simulink model "TCT_long_wide_PVArray_PartialShading"  (R2016b)
settings: Solver=ode23tb  StartTime=0.0  StopTime=5  FixedStep=Ts_Power  RelTol=1e-4
PreLoadFcn:
  | Ts_Power=50e-6;
  | Slope_Vdc=1;
InitFcn:
  | Ts_Power=50e-6;
  | Tc=1e-5;%break algebraic loop time constant
  | BlockName=[gcs,'/PV cells 1-20'];
  | ModuleName=get_param(BlockName,'ModuleName');
  | Voc1=str2num(get_param(BlockName,'Voc'));
  | Nser1=str2num(get_param(BlockName,'Nser'));
  | Slope_Vdc=Nser1*Voc1;
StopFcn:
  | if exist('I','var') && exist('V','var')
  |    figure(1)
  |    clf
  |    n=find(I>=0);
  |    n=n(end);
  |    Vglobal=V(1:n);
  |    Iglobal=I(1:n);
  | 
  | 
  |    Pglobal=Vglobal.*Iglobal;
  |    n=find(Pglobal==max(Pglobal));
  |    Pmax=Pglobal(n);
  |    Vmp=Vglobal(n);
  |    Imp=Iglobal(n);
  | 
  | 
  |    subplot(211)
  |    plot(Vglobal, Iglobal,Vmp,Imp,'or')
  |    ylabel('Current (A)')
  |    title(sprintf('Global I-V & P-V characteristics\n %s' ,ModuleName))
  | 
  | 
  |    subplot(212)
  |    plot(Vglobal, Pglobal,Vmp,Pmax,'or')
  |    ylabel('Power (W)')
  |    xlabel('Voltage (V)')
  | end
libraries: powerlib x29, re_lib x25, simulink x1
Description:
  | Copyright 2008-2016 The MathWorks, Inc.
settings Model: Creator=MathWorks  LastModifiedBy=Gehaha
settings SolverCC: AlgebraicLoopSolver=LineSearch
settings DataIOCC: LimitDataPoints=on  SaveFormat=Array  SignalLoggingSaveFormat=ModelDataLogs
settings OptimizationCC: ExpressionDepthLimit=2147483647  LifeSpan=inf
settings DebuggingCC: UnderspecifiedInitializationDetection=Classic  MergeDetectMultiDrivingBlocksExec=none  SolverPrmCheckMsg=warning  FcnCallInpInsideContextMsg=warning  AllowSymbolicDim=off  StateNameClashWarn=warning  SFUnexpectedBacktrackingDiag=warning  SFNoUnconditionalDefaultTransitionDiag=warning  SFExecutionAtInitializationDiag=none
settings HardwareCC: ProdBitPerPointer=32  ProdBitPerSizeT=32  ProdBitPerPtrDiffT=32  ProdLargestAtomicFloat=None  ProdIntDivRoundTo=Undefined  ProdEndianess=Unspecified  ProdWordSize=32  ProdHWDeviceType=32-bit Generic
settings ModelReferenceCC: PropagateSignalLabelsOutOfModel=off
settings GRTTargetCC: TargetLangStandard=C89/C90 (ANSI)  GeneratePreprocessorConditionals=Disable all  CombineOutputUpdateFcns=off  GRTInterface=on
settings ConfigComp: CovMetricSettings=dw  CovHtmlReporting=on  CovSaveCumulativeToWorkspaceVar=on  CovSaveSingleToWorkspaceVar=on  CovExternalEMLEnable=off  CovSFcnEnable=off

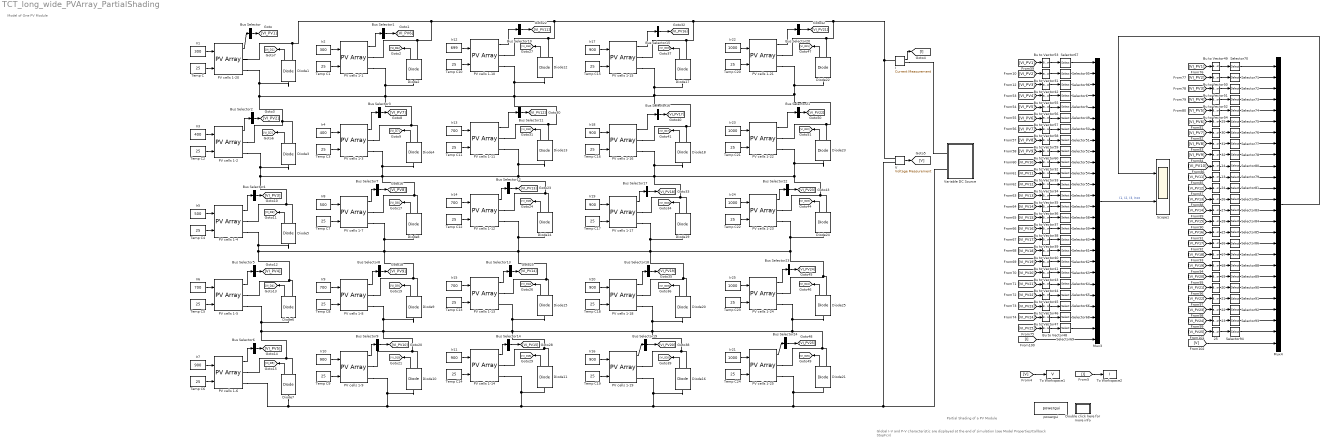
== system TCT_long_wide_PVArray_PartialShading ==
  note: Global I-V and P-V characteristic are displayed at the end of simulation
      | (see Model Properties/Callback StopFcn)
  note: Partial Shading of a PV Module
  note: Model of One PV Module
  {13..32} (20 alike) : BusToVector
  Bu to Vector{31..60} (30 alike) : BusToVector
  Bus Selector{,1..24} (25 alike) : BusSelector  OutputSignals=V_PV,I_PV  OutputAsBus=on
  Diode{1..25} (25 alike) : powerlib/Power Electronics/Diode  Ron=0.001  Lon=0  Vf=0.7  IC=0  UseSnubber=off  Rs=1e5*inf  Cs=inf  Measurements=on
  Double click here for more info : Subsystem
      settings: OpenFcn=showdemo(bdroot(gcb))
      mask Display: disp('?')
  I : powerlib/Measurements/Current Measurement  PhasorSimulation=off  OutputType=Complex  PSBequivalent=0
  Ir1 : Constant  Value=300
  Ir{7,10..11,16..20} (8 alike) : Constant  Value=900
  Ir12 : Constant  Value=699
  Ir{6,9,13..15} (5 alike) : Constant  Value=700
  Ir2 : Constant  Value=300
  Ir{21..25} (5 alike) : Constant  Value=1000
  Ir3 : Constant  Value=400
  Ir4 : Constant  Value=400
  Ir5 : Constant  Value=500
  Ir8 : Constant  Value=500
  Mux3 : Mux  Inputs=26
  Mux4 : Mux  Inputs=26
  PV cells 1-{1..25} (25 alike) : re_lib/Solar/PV Array  Npar=1  Nser=1  PlotType=array @ 25 deg.C & specified irradiances  S_vec="[ 1000  500  100 ]"  Temp_C_vec="[ 45 25  ]"  ModuleName=User-defined  PlotWhenSelected=off  Pm=83.2824  Ncell=60/3  Voc=37.92*20/60  Isc=8.62  Vm=30.96*20/60  Im=8.07  beta_Voc_pc=-0.33969  alpha_Isc_pc=0.063701  beta_Voc=-0.042937  alpha_Isc=0.005491  IL=8.6307  I0=1.4176e-10  nI=0.99132  Rsh=82.1161  Rs=0.098625  BAL=on  Tc=Tc  Tfilter=5e-5
  Scope1 : Scope  NumInputPorts=2
  Selector{6,9,49..69,95..96} (25 alike) : Selector  InputPortWidth=2  IndexOptions=Index vector (dialog)  Indices=[2]  OutputSizes=1
  Selector{70..94} (25 alike) : Selector  InputPortWidth=2  IndexOptions=Index vector (dialog)  Indices=[1]  OutputSizes=1
  Temp C{,1..24} (25 alike) : Constant  Value=25
  To Workspace1 : ToWorkspace  VariableName=V  SampleTime=1e-3
  To Workspace2 : ToWorkspace  VariableName=I  SampleTime=1e-3
  V : powerlib/Measurements/Voltage Measurement  PhasorSimulation=off  OutputType=Complex  PSBequivalent=0
  Variable DC Source : Subsystem
  powergui : powerlib/powergui  Priority=1  SimulationMode=Continuous  SolverType=Tustin/Backward Euler (TBE)  SampleTime=Ts_Power*0 + 20e-6  frequency=60  SPID=off  DisableSnubberDevices=on  DisableRonSwitches=off  DisableVfSwitches=off  SwTol=0  DisplayEquations=off  Interpol=off  ExternalGateDelay=off  methode=off  Ts=0  FunctionMessages=off  echomessages=off  HookPort=off  EnableUseOfTLC=off  x0status=blocks  frequencyindice=0  Pbase=100e6  ErrMax=1e-4  Iterations=50  UnitsV=kV  UnitsW=MW  buscounter=0  RestoreLinks=warning  ResistiveCurrentMeasurement=off  Frange=[0:2:500]  Ylog=off  Xlog=on  ShowGrid=off  save=off  variable=ZData  structure=0  ZoomFFT=on  StartTime=0.0  cycles=1  DisplayStyle=1  fundamental=60  FreqAxis=off  MaxFrequency=1000  frequencyindicesteady=1  RmsSteady=1  display=off
  wires:
  Ir1/1 -> PV cells 1-20/1
  Temp C/1 -> PV cells 1-20/2
  I/1 -> [I]
  V/1 -> [V]
  Diode1/1 -> [VI_D1]
  PV cells 1-20/1 -> Bus Selector/1
  Bus Selector/1 -> [VI_PV1]
  [V] -> To Workspace1/1
  [I] -> To Workspace2/1
  Ir2/1 -> PV cells 1-1/1
  Temp C1/1 -> PV cells 1-1/2
  Diode2/1 -> [VI_D6]
  PV cells 1-1/1 -> Bus Selector1/1
  Bus Selector1/1 -> [VI_PV6]
  Ir3/1 -> PV cells 1-2/1
  Temp C2/1 -> PV cells 1-2/2
  Diode3/1 -> [VI_D2]
  PV cells 1-2/1 -> Bus Selector2/1
  Bus Selector2/1 -> [VI_PV2]
  Ir4/1 -> PV cells 1-3/1
  Temp C3/1 -> PV cells 1-3/2
  Diode4/1 -> [VI_D7]
  PV cells 1-3/1 -> Bus Selector3/1
  Bus Selector3/1 -> [VI_PV7]
  Ir5/1 -> PV cells 1-4/1
  Temp C4/1 -> PV cells 1-4/2
  Diode5/1 -> [VI_D3]
  PV cells 1-4/1 -> Bus Selector4/1
  Bus Selector4/1 -> [VI_PV3]
  Ir6/1 -> PV cells 1-5/1
  Temp C5/1 -> PV cells 1-5/2
  Diode6/1 -> [VI_D4]
  PV cells 1-5/1 -> Bus Selector5/1
  Bus Selector5/1 -> [VI_PV4]
  Ir7/1 -> PV cells 1-6/1
  Temp C6/1 -> PV cells 1-6/2
  Diode7/1 -> [VI_D5]
  PV cells 1-6/1 -> Bus Selector6/1
  Bus Selector6/1 -> [VI_PV5]
  Ir8/1 -> PV cells 1-7/1
  Temp C7/1 -> PV cells 1-7/2
  Diode8/1 -> [VI_D8]
  PV cells 1-7/1 -> Bus Selector7/1
  Bus Selector7/1 -> [VI_PV8]
  Ir9/1 -> PV cells 1-8/1
  Temp C8/1 -> PV cells 1-8/2
  Diode9/1 -> [VI_D9]
  PV cells 1-8/1 -> Bus Selector8/1
  Bus Selector8/1 -> [VI_PV9]
  Ir10/1 -> PV cells 1-9/1
  Temp C9/1 -> PV cells 1-9/2
  Diode10/1 -> [VI_D10]
  PV cells 1-9/1 -> Bus Selector9/1
  Bus Selector9/1 -> [VI_PV10]
  Ir12/1 -> PV cells 1-10/1
  Temp C10/1 -> PV cells 1-10/2
  Diode12/1 -> [VI_D11]
  PV cells 1-10/1 -> Bus Selector10/1
  Bus Selector10/1 -> [VI_PV11]
  Ir13/1 -> PV cells 1-11/1
  Temp C11/1 -> PV cells 1-11/2
  Diode13/1 -> [VI_D12]
  PV cells 1-11/1 -> Bus Selector11/1
  Bus Selector11/1 -> [VI_PV12]
  Ir14/1 -> PV cells 1-12/1
  Temp C12/1 -> PV cells 1-12/2
  Diode14/1 -> [VI_D13]
  PV cells 1-12/1 -> Bus Selector12/1
  Bus Selector12/1 -> [VI_PV13]
  Ir15/1 -> PV cells 1-13/1
  Temp C13/1 -> PV cells 1-13/2
  Diode15/1 -> [VI_D14]
  PV cells 1-13/1 -> Bus Selector13/1
  Bus Selector13/1 -> [VI_PV14]
  Ir11/1 -> PV cells 1-14/1
  Temp C14/1 -> PV cells 1-14/2
  Diode11/1 -> [VI_D15]
  PV cells 1-14/1 -> Bus Selector14/1
  Bus Selector14/1 -> [VI_PV15]
  Ir17/1 -> PV cells 1-15/1
  Temp C15/1 -> PV cells 1-15/2
  Diode17/1 -> [VI_D16]
  PV cells 1-15/1 -> Bus Selector15/1
  Bus Selector15/1 -> [VI_PV16]
  Ir18/1 -> PV cells 1-16/1
  Temp C16/1 -> PV cells 1-16/2
  Diode18/1 -> [VI_D17]
  PV cells 1-16/1 -> Bus Selector16/1
  Bus Selector16/1 -> [VI_PV17]
  Ir19/1 -> PV cells 1-17/1
  Temp C17/1 -> PV cells 1-17/2
  Diode19/1 -> [VI_D18]
  PV cells 1-17/1 -> Bus Selector17/1
  Bus Selector17/1 -> [VI_PV18]
  Ir20/1 -> PV cells 1-18/1
  Temp C18/1 -> PV cells 1-18/2
  Diode20/1 -> [VI_D19]
  PV cells 1-18/1 -> Bus Selector18/1
  Bus Selector18/1 -> [VI_PV19]
  Ir16/1 -> PV cells 1-19/1
  Temp C19/1 -> PV cells 1-19/2
  Diode16/1 -> [VI_D20]
  PV cells 1-19/1 -> Bus Selector19/1
  Bus Selector19/1 -> [VI_PV20]
  Ir22/1 -> PV cells 1-21/1
  Temp C20/1 -> PV cells 1-21/2
  Diode22/1 -> [VI_D21]
  PV cells 1-21/1 -> Bus Selector20/1
  Bus Selector20/1 -> [VI_PV21]
  Ir23/1 -> PV cells 1-22/1
  Temp C21/1 -> PV cells 1-22/2
  Diode23/1 -> [VI_D22]
  PV cells 1-22/1 -> Bus Selector21/1
  Bus Selector21/1 -> [VI_PV22]
  Ir24/1 -> PV cells 1-23/1
  Temp C22/1 -> PV cells 1-23/2
  Diode24/1 -> [VI_D23]
  PV cells 1-23/1 -> Bus Selector22/1
  Bus Selector22/1 -> [VI_PV23]
  Ir25/1 -> PV cells 1-24/1
  Temp C23/1 -> PV cells 1-24/2
  Diode25/1 -> [VI_D24]
  PV cells 1-24/1 -> Bus Selector23/1
  Bus Selector23/1 -> [VI_PV24]
  Ir21/1 -> PV cells 1-25/1
  Temp C24/1 -> PV cells 1-25/2
  Diode21/1 -> [VI_D25]
  PV cells 1-25/1 -> Bus Selector24/1
  Bus Selector24/1 -> [VI_PV25]
  Mux3/1 -> Scope1/2  "I1, I2, I3, Itot"
  [VI_PV1] -> Bu to Vector53/1
  Selector67/1 -> Mux3/1
  Bu to Vector53/1 -> Selector67/1
  [I] -> Mux3/26
  Selector95/1 -> Mux3/2
  Selector96/1 -> Mux3/3
  Selector6/1 -> Mux3/4
  Selector9/1 -> Mux3/5
  Selector49/1 -> Mux3/6
  Selector50/1 -> Mux3/7
  [VI_PV2] -> Bu to Vector31/1
  Bu to Vector31/1 -> Selector95/1
  [VI_PV3] -> Bu to Vector42/1
  Bu to Vector42/1 -> Selector96/1
  [VI_PV4] -> Bu to Vector55/1
  Bu to Vector55/1 -> Selector6/1
  [VI_PV5] -> Bu to Vector56/1
  Bu to Vector56/1 -> Selector9/1
  [VI_PV6] -> Bu to Vector57/1
  Bu to Vector57/1 -> Selector49/1
  [VI_PV7] -> Bu to Vector58/1
  Bu to Vector58/1 -> Selector50/1
  [VI_PV8] -> Bu to Vector59/1
  Bu to Vector59/1 -> Selector51/1
  Selector51/1 -> Mux3/8
  [VI_PV9] -> Bu to Vector60/1
  Bu to Vector60/1 -> Selector52/1
  Selector52/1 -> Mux3/9
  [VI_PV10] -> Bu to Vector32/1
  Bu to Vector32/1 -> Selector53/1
  Selector53/1 -> Mux3/10
  [VI_PV11] -> Bu to Vector33/1
  Bu to Vector33/1 -> Selector54/1
  Selector54/1 -> Mux3/11
  [VI_PV12] -> Bu to Vector34/1
  Bu to Vector34/1 -> Selector55/1
  Selector55/1 -> Mux3/12
  [VI_PV13] -> Bu to Vector35/1
  Bu to Vector35/1 -> Selector56/1
  Selector56/1 -> Mux3/13
  [VI_PV14] -> Bu to Vector36/1
  Bu to Vector36/1 -> Selector57/1
  Selector57/1 -> Mux3/14
  [VI_PV15] -> Bu to Vector37/1
  Bu to Vector37/1 -> Selector58/1
  Selector58/1 -> Mux3/15
  [VI_PV16] -> Bu to Vector38/1
  Bu to Vector38/1 -> Selector59/1
  Selector59/1 -> Mux3/16
  [VI_PV17] -> Bu to Vector39/1
  Bu to Vector39/1 -> Selector60/1
  Selector60/1 -> Mux3/17
  [VI_PV18] -> Bu to Vector40/1
  Bu to Vector40/1 -> Selector61/1
  Selector61/1 -> Mux3/18
  [VI_PV19] -> Bu to Vector41/1
  Bu to Vector41/1 -> Selector62/1
  Selector62/1 -> Mux3/19
  [VI_PV20] -> Bu to Vector43/1
  Bu to Vector43/1 -> Selector63/1
  Selector63/1 -> Mux3/20
  [VI_PV21] -> Bu to Vector44/1
  Bu to Vector44/1 -> Selector64/1
  Selector64/1 -> Mux3/21
  [VI_PV22] -> Bu to Vector45/1
  Bu to Vector45/1 -> Selector65/1
  Selector65/1 -> Mux3/22
  [VI_PV23] -> Bu to Vector46/1
  Bu to Vector46/1 -> Selector66/1
  Selector66/1 -> Mux3/23
  [VI_PV24] -> Bu to Vector47/1
  Bu to Vector47/1 -> Selector68/1
  Selector68/1 -> Mux3/24
  [VI_PV25] -> Bu to Vector48/1
  Bu to Vector48/1 -> Selector69/1
  Selector69/1 -> Mux3/25
  [VI_PV1] -> Bu to Vector49/1
  Selector70/1 -> Mux4/1
  Bu to Vector49/1 -> Selector70/1
  Selector71/1 -> Mux4/2
  [VI_PV2] -> Bu to Vector50/1
  Bu to Vector50/1 -> Selector71/1
  Selector72/1 -> Mux4/3
  [VI_PV3] -> Bu to Vector51/1
  Bu to Vector51/1 -> Selector72/1
  Selector73/1 -> Mux4/4
  [VI_PV4] -> Bu to Vector52/1
  Bu to Vector52/1 -> Selector73/1
  [VI_PV5] -> Bu to Vector54/1
  Bu to Vector54/1 -> Selector74/1
  Selector74/1 -> Mux4/5
  Selector75/1 -> Mux4/6
  [VI_PV6] -> 29/1
  29/1 -> Selector75/1
  Selector76/1 -> Mux4/7
  [VI_PV7] -> 30/1
  30/1 -> Selector76/1
  Selector77/1 -> Mux4/8
  [VI_PV8] -> 31/1
  31/1 -> Selector77/1
  [VI_PV9] -> 32/1
  32/1 -> Selector78/1
  Selector78/1 -> Mux4/9
  [VI_PV10] -> 14/1
  14/1 -> Selector80/1
  Selector80/1 -> Mux4/10
  [VI_PV11] -> 13/1
  13/1 -> Selector79/1
  Selector79/1 -> Mux4/11
  [VI_PV12] -> 24/1
  24/1 -> Selector81/1
  Selector81/1 -> Mux4/12
  [VI_PV13] -> 26/1
  26/1 -> Selector82/1
  Selector82/1 -> Mux4/13
  [VI_PV14] -> 27/1
  27/1 -> Selector83/1
  Selector83/1 -> Mux4/14
  [VI_PV15] -> 28/1
  28/1 -> Selector84/1
  Selector84/1 -> Mux4/15
  [VI_PV16] -> 15/1
  15/1 -> Selector85/1
  Selector85/1 -> Mux4/16
  [VI_PV17] -> 16/1
  16/1 -> Selector86/1
  Selector86/1 -> Mux4/17
  [VI_PV18] -> 17/1
  17/1 -> Selector87/1
  Selector87/1 -> Mux4/18
  [VI_PV19] -> 18/1
  18/1 -> Selector88/1
  Selector88/1 -> Mux4/19
  [VI_PV20] -> 19/1
  19/1 -> Selector89/1
  Selector89/1 -> Mux4/20
  [VI_PV21] -> 20/1
  20/1 -> Selector90/1
  Selector90/1 -> Mux4/21
  [VI_PV22] -> 21/1
  21/1 -> Selector91/1
  Selector91/1 -> Mux4/22
  [VI_PV23] -> 22/1
  22/1 -> Selector92/1
  Selector92/1 -> Mux4/23
  [VI_PV24] -> 23/1
  23/1 -> Selector93/1
  Selector93/1 -> Mux4/24
  [VI_PV25] -> 25/1
  25/1 -> Selector94/1
  Selector94/1 -> Mux4/25
  [V] -> Mux4/26
  Mux4/1 -> Scope1/1
  connections:
  I/RConn1 -- Variable DC Source/LConn1
  Diode22/RConn1 -- I/LConn1 -- V/LConn1 -- PV cells 1-15/RConn1 -- Diode17/RConn1 -- Diode12/RConn1 -- PV cells 1-10/RConn1 -- Diode2/RConn1 -- PV cells 1-1/RConn1 -- Diode1/RConn1 -- PV cells 1-20/RConn1 -- PV cells 1-21/RConn1
  PV cells 1-25/RConn2 -- V/LConn2 -- Variable DC Source/LConn2 -- PV cells 1-6/RConn2 -- Diode7/LConn1 -- Diode10/LConn1 -- PV cells 1-9/RConn2 -- Diode11/LConn1 -- PV cells 1-14/RConn2 -- Diode16/LConn1 -- PV cells 1-19/RConn2 -- Diode21/LConn1
  PV cells 1-24/RConn2 -- Diode25/LConn1 -- Diode21/RConn1 -- PV cells 1-25/RConn1 -- Diode16/RConn1 -- PV cells 1-19/RConn1 -- PV cells 1-5/RConn2 -- Diode6/LConn1 -- Diode7/RConn1 -- PV cells 1-6/RConn1 -- Diode9/LConn1 -- PV cells 1-8/RConn2 -- Diode10/RConn1 -- PV cells 1-9/RConn1 -- Diode11/RConn1 -- PV cells 1-14/RConn1 -- Diode15/LConn1 -- PV cells 1-13/RConn2 -- Diode20/LConn1 -- PV cells 1-18/RConn2
  PV cells 1-21/RConn2 -- Diode22/LConn1 -- Diode18/RConn1 -- PV cells 1-16/RConn1 -- PV cells 1-20/RConn2 -- Diode1/LConn1 -- Diode3/RConn1 -- PV cells 1-2/RConn1 -- Diode2/LConn1 -- PV cells 1-1/RConn2 -- Diode4/RConn1 -- PV cells 1-3/RConn1 -- Diode13/RConn1 -- PV cells 1-11/RConn1 -- Diode12/LConn1 -- PV cells 1-10/RConn2 -- Diode17/LConn1 -- PV cells 1-15/RConn2 -- Diode23/RConn1 -- PV cells 1-22/RConn1
  PV cells 1-22/RConn2 -- Diode23/LConn1 -- Diode24/RConn1 -- PV cells 1-23/RConn1 -- PV cells 1-2/RConn2 -- Diode3/LConn1 -- Diode5/RConn1 -- PV cells 1-4/RConn1 -- PV cells 1-7/RConn1 -- Diode8/RConn1 -- Diode4/LConn1 -- PV cells 1-3/RConn2 -- Diode14/RConn1 -- PV cells 1-12/RConn1 -- Diode13/LConn1 -- PV cells 1-11/RConn2 -- Diode19/RConn1 -- PV cells 1-17/RConn1 -- Diode18/LConn1 -- PV cells 1-16/RConn2
  PV cells 1-23/RConn2 -- Diode24/LConn1 -- PV cells 1-24/RConn1 -- Diode25/RConn1 -- PV cells 1-4/RConn2 -- Diode5/LConn1 -- Diode6/RConn1 -- PV cells 1-5/RConn1 -- Diode9/RConn1 -- PV cells 1-8/RConn1 -- Diode8/LConn1 -- PV cells 1-7/RConn2 -- Diode14/LConn1 -- PV cells 1-12/RConn2 -- Diode15/RConn1 -- PV cells 1-13/RConn1 -- PV cells 1-18/RConn1 -- Diode20/RConn1 -- Diode19/LConn1 -- PV cells 1-17/RConn2

== system TCT_long_wide_PVArray_PartialShading/Double click here for more info ==

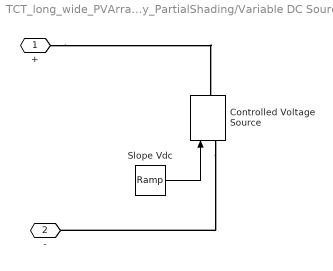
== system TCT_long_wide_PVArray_PartialShading/Variable DC Source ==
  Controlled Voltage Source : powerlib/Electrical Sources/Controlled Voltage Source  Initialize=on  Source_Type=AC  Amplitude=0  Phase=0  Frequency=0  Measurements=None
  Slope Vdc : simulink/Sources/Ramp  slope=Slope_Vdc  start=0  X0=0
  + : PMIOPort  Port=1  Side=Left
  - : PMIOPort  Port=2  Side=Left
  wires:
  Slope Vdc/1 -> Controlled Voltage Source/1
  connections:
  Controlled Voltage Source/LConn1 -- -/RConn1
  +/RConn1 -- Controlled Voltage Source/RConn1
